simulink library "cart2cyl"  (R2018b)
settings: Solver=VariableStepAuto  StartTime=0.0  StopTime=10.0  RelTol=1e-3
settings Model: Creator=BI28030  LastModifiedBy=BI28030

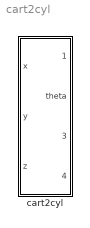
== system cart2cyl ==
  cart2cyl : Subsystem  mask(cart2cyl){}
      mask help: cart2cyl

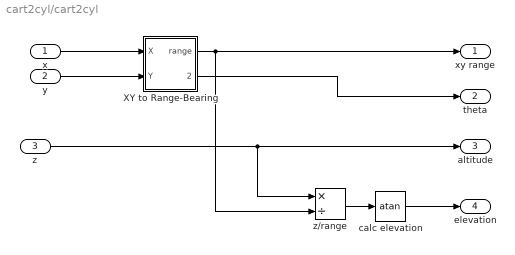
== system cart2cyl/cart2cyl ==
  x : Inport
  y : Inport  Port=2
  z : Inport  Port=3
  XY to Range-Bearing : Subsystem  mask(xy2rtheta){}
      mask help:
      | Vector transformation from cartesian to polar coordinates.
      | input:   [x, y]
      | output: [r, theta]
      |
      | r = hypot(x,y));
      | theta = atan2(y,x);
      mask Help: Use "Look under mask" to see the implementation, done in Simulink blocks.
      mask Display: plot(0,0,100,100,[24,20,15,20,20],[85,95,85,95,20],[80,20,95,85,95,85],[70,20,20,15,20,24],[56,56,55,52,50,46],[20,26,31,35,38,42])
  calc elevation : Trigonometry  Operator=atan
  z/range : Product  Inputs=*/
  xy range : Outport
  theta : Outport  Port=2
  altitude : Outport  Port=3
  elevation : Outport  Port=4
  wires:
  z/range/1 -> calc elevation/1
  calc elevation/1 -> elevation/1
  XY to Range-Bearing/2(bearing) -> theta/1
  XY to Range-Bearing/1(range) -> xy range/1, z/range/2
  y/1 -> XY to Range-Bearing/2(Y)
  x/1 -> XY to Range-Bearing/1(X)
  z/1 -> altitude/1, z/range/1

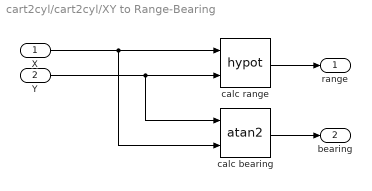
== system cart2cyl/cart2cyl/XY to Range-Bearing ==
  X : Inport
  Y : Inport  Port=2
  calc bearing : Trigonometry  Operator=atan2
  calc range : Math  Operator=hypot  SaturateOnIntegerOverflow=on
  range : Outport
  bearing : Outport  Port=2
  wires:
  calc bearing/1 -> bearing/1
  calc range/1 -> range/1
  Y/1 -> calc range/2, calc bearing/1
  X/1 -> calc range/1, calc bearing/2
